simulink model "rigidBody2d03v"  (Simulink 7.5)
settings: Solver=ode45  StartTime=0.0  StopTime=2  RelTol=1e-4
values from neighbouring files (symbols this model uses):
  c = 1000    [runModel03v.m]    (also in runModel04v.m = 5000)
  dy = 0    [runModel03v.m]    (also in runModel04v.m)
  dyt1 = .2    (= 0.2)    [runModel03v.m]    (also in runModel04v.m = 1000)
  dyt2 = .2 + L/v0    (= 0.231666666667)    [runModel03v.m]    (also in runModel04v.m = 1000)
  FB1t = .2    (= 0.2)    [runModel03v.m]
  FB1x = -1600    [runModel03v.m]
  FB2 = [-1600 0]    [runModel03v.m]
  FD = [-645 0]    [runModel03v.m]    (also in runModel04v.m)
  FE1 = [120 0]    [runModel03v.m]    (also in runModel04v.m)
  FE2t = 1000    [runModel03v.m]    (also in runModel04v.m = 10000)
  FE2x = 120    [runModel03v.m]    (also in runModel04v.m)
  I = 1/4*m*R^2 + 1/12*m*L^2    (= 405.066666667)    [runModel03v.m]    (also in runModel04v.m)
  k = 111000*2    (= 222000)    [runModel03v.m]    (also in runModel04v.m)
  L = 3.8    [runModel03v.m]    (also in runModel04v.m)
  m = 320    [runModel03v.m]    (also in runModel04v.m)
  rB1 = [0 0.5]    [runModel03v.m]    (also in runModel04v.m)
  rB2 = [0 -0.5]    [runModel03v.m]    (also in runModel04v.m)
  rDx = 0    [runModel03v.m]    (also in runModel04v.m)
  rE1 = [0 0.5]    [runModel03v.m]    (also in runModel04v.m)
  rE2 = [0 -0.5]    [runModel03v.m]    (also in runModel04v.m)
  rS1 = [-1.9 0]    [runModel03v.m]    (also in runModel04v.m)
  rS2 = [1.9 0]    [runModel03v.m]    (also in runModel04v.m)
  v0 = 120    [runModel03v.m]    (also in runModel04v.m)
settings Model: Creator=aaron  LastModifiedBy=aaron
settings DebuggingCC: SolverPrmCheckMsg=none

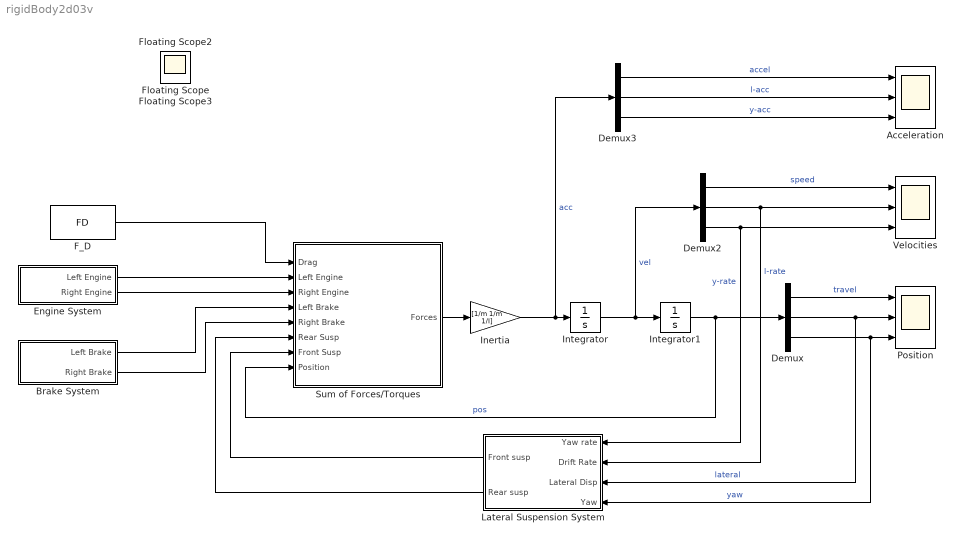
== system rigidBody2d03v ==
  Acceleration : Scope  NumInputPorts=3
      settings: TimeRange=2  YMin=1~-1~-1  YMax=3.5~1~1  SaveName=position3
  Brake System : Subsystem
  Demux : Demux  Outputs=3
  Demux2 : Demux  Outputs=3
  Demux3 : Demux  Outputs=3
  Engine System : Subsystem
  F_D : Constant  Value=FD  OutDataType=fixdt(1, 16)  OutScaling=2^0
  Inertia : Gain  Gain=[1/m 1/m 1/I]  ParameterDataType=fixdt(1, 16)  ParameterScaling=2^0  OutDataType=fixdt(1, 16)  OutScaling=2^0
  Integrator : Integrator  InitialCondition=[v0 0 0]
  Integrator1 : Integrator  InitialCondition=[0 0 0]
  Lateral Suspension System : Subsystem
  Position : Scope  NumInputPorts=3
      settings: YMin=-1.5e+007~-52.5~-0.7  YMax=0~2.5~0.05  SaveName=position
  Sum of Forces/Torques : Subsystem
  Velocities : Scope  NumInputPorts=3
      settings: YMin=-5~-5~-5  YMax=5~5~5  SaveName=position2
  Floating Scope : Scope
      settings: Floating=on
  Floating Scope2 : Scope
      settings: Floating=on  SaveName=ScopeData2
  Floating Scope3 : Scope
      settings: Floating=on  SaveName=ScopeData3
  wires:
  Integrator/1 -> Integrator1/1, Demux2/1  "vel"
  Inertia/1 -> Demux3/1, Integrator/1  "acc"
  Sum of Forces/Torques/1(Forces) -> Inertia/1
  Integrator1/1 -> Demux/1, Sum of Forces/Torques/8(Position)  "pos"
  Demux/1 -> Position/1  "travel"
  Demux/2 -> Position/2, Lateral Suspension System/3(Lateral Disp)  "lateral"
  Demux/3 -> Position/3, Lateral Suspension System/4(Yaw)  "yaw"
  Demux2/1 -> Velocities/1  "speed"
  Demux2/2 -> Velocities/2, Lateral Suspension System/2(Drift Rate)  "l-rate"
  Demux2/3 -> Velocities/3, Lateral Suspension System/1(Yaw rate)  "y-rate"
  Demux3/1 -> Acceleration/1  "accel"
  Demux3/2 -> Acceleration/2  "l-acc"
  Demux3/3 -> Acceleration/3  "y-acc"
  Engine System/1(Left Engine) -> Sum of Forces/Torques/2(Left Engine)
  Lateral Suspension System/1(Front susp) -> Sum of Forces/Torques/7(Front Susp)
  Lateral Suspension System/2(Rear susp) -> Sum of Forces/Torques/6(Rear Susp)
  F_D/1 -> Sum of Forces/Torques/1(Drag)
  Engine System/2(Right Engine) -> Sum of Forces/Torques/3(Right Engine)
  Brake System/1(Left Brake) -> Sum of Forces/Torques/4(Left Brake)
  Brake System/2(Right Brake) -> Sum of Forces/Torques/5(Right Brake)

== system rigidBody2d03v/Brake System ==
  F_B1y : Constant  Value=0  OutDataType=fixdt(1, 16)  OutScaling=2^0
  F_B2 : Constant  Value=FB2  OutDataType=fixdt(1, 16)  OutScaling=2^0
  Mux : Mux  Inputs=2
  Step : Step  Time=FB1t  Before=FB1x  After=0  SampleTime=0
  Left Brake : Outport
  Right Brake : Outport  Port=2
  wires:
  Step/1 -> Mux/1  "forceX"
  F_B1y/1 -> Mux/2  "forceY"
  F_B2/1 -> Right Brake/1
  Mux/1 -> Left Brake/1

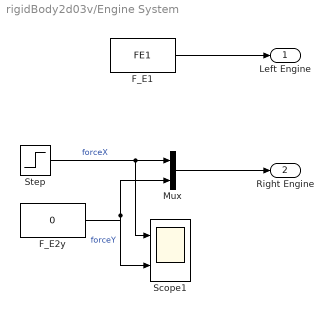
== system rigidBody2d03v/Engine System ==
  F_E1 : Constant  Value=FE1  OutDataType=fixdt(1, 16)  OutScaling=2^0
  F_E2y : Constant  Value=0  OutDataType=fixdt(1, 16)  OutScaling=2^0
  Mux : Mux  Inputs=2
  Scope1 : Scope  NumInputPorts=2
      settings: YMin=-5~-5  YMax=5~5  SaveName=engineErr
  Step : Step  Time=FE2t  Before=FE2x  After=0  SampleTime=0
  Left Engine : Outport
  Right Engine : Outport  Port=2
  wires:
  Step/1 -> Mux/1, Scope1/1  "forceX"
  F_E2y/1 -> Mux/2, Scope1/2  "forceY"
  F_E1/1 -> Left Engine/1
  Mux/1 -> Right Engine/1

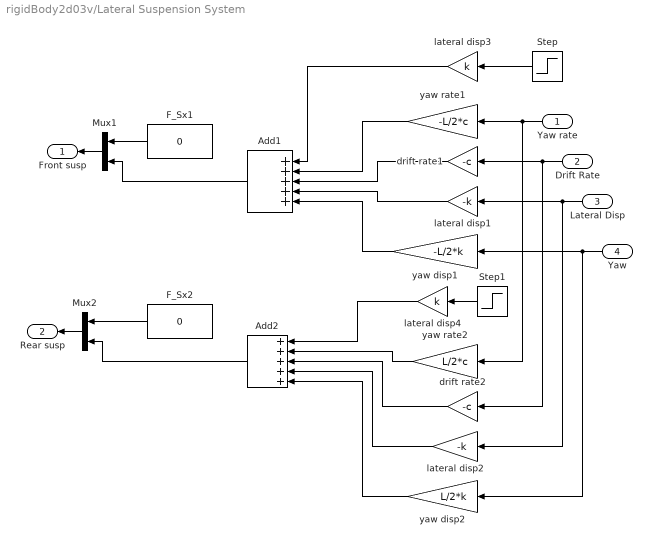
== system rigidBody2d03v/Lateral Suspension System ==
  Yaw rate : Inport
  Drift Rate : Inport  Port=2
  Lateral Disp : Inport  Port=3
  Yaw : Inport  Port=4
  Add1 : Sum  Inputs=+++++  OutDataType=fixdt(1, 16)  OutScaling=2^-10
  Add2 : Sum  Inputs=+++++  OutDataType=fixdt(1, 16)  OutScaling=2^-10
  F_Sx1 : Constant  Value=0  OutDataType=fixdt(1, 16)  OutScaling=2^0
  F_Sx2 : Constant  Value=0  OutDataType=fixdt(1, 16)  OutScaling=2^0
  Mux1 : Mux  Inputs=2
  Mux2 : Mux  Inputs=2
  Step : Step  Time=dyt1  After=dy  SampleTime=0
  Step1 : Step  Time=dyt2  After=dy  SampleTime=0
  drift rate1 : Gain  Gain=-c  ParameterDataType=fixdt(1, 16)  ParameterScaling=2^0  OutDataType=fixdt(1, 16)  OutScaling=2^0
  drift rate2 : Gain  Gain=-c  ParameterDataType=fixdt(1, 16)  ParameterScaling=2^0  OutDataType=fixdt(1, 16)  OutScaling=2^0
  lateral disp1 : Gain  Gain=-k  ParameterDataType=fixdt(1, 16)  ParameterScaling=2^0  OutDataType=fixdt(1, 16)  OutScaling=2^0
  lateral disp2 : Gain  Gain=-k  ParameterDataType=fixdt(1, 16)  ParameterScaling=2^0  OutDataType=fixdt(1, 16)  OutScaling=2^0
  lateral disp3 : Gain  Gain=k  ParameterDataType=fixdt(1, 16)  ParameterScaling=2^0  OutDataType=fixdt(1, 16)  OutScaling=2^0
  lateral disp4 : Gain  Gain=k  ParameterDataType=fixdt(1, 16)  ParameterScaling=2^0  OutDataType=fixdt(1, 16)  OutScaling=2^0
  yaw disp1 : Gain  Gain=-L/2*k  ParameterDataType=fixdt(1, 16)  ParameterScaling=2^0  OutDataType=fixdt(1, 16)  OutScaling=2^0
  yaw disp2 : Gain  Gain=L/2*k  ParameterDataType=fixdt(1, 16)  ParameterScaling=2^0  OutDataType=fixdt(1, 16)  OutScaling=2^0
  yaw rate1 : Gain  Gain=-L/2*c  ParameterDataType=fixdt(1, 16)  ParameterScaling=2^0  OutDataType=fixdt(1, 16)  OutScaling=2^0
  yaw rate2 : Gain  Gain=L/2*c  ParameterDataType=fixdt(1, 16)  ParameterScaling=2^0  OutDataType=fixdt(1, 16)  OutScaling=2^0
  Front susp : Outport
  Rear susp : Outport  Port=2
  wires:
  F_Sx1/1 -> Mux1/1
  Add1/1 -> Mux1/2
  F_Sx2/1 -> Mux2/1
  Add2/1 -> Mux2/2
  lateral disp1/1 -> Add1/4
  lateral disp2/1 -> Add2/4
  drift rate2/1 -> Add2/3
  drift rate1/1 -> Add1/3
  yaw disp2/1 -> Add2/5
  yaw disp1/1 -> Add1/5
  yaw rate2/1 -> Add2/2
  yaw rate1/1 -> Add1/2
  Yaw rate/1 -> yaw rate1/1, yaw rate2/1
  Drift Rate/1 -> drift rate1/1, drift rate2/1
  Lateral Disp/1 -> lateral disp1/1, lateral disp2/1
  Yaw/1 -> yaw disp1/1, yaw disp2/1
  Mux1/1 -> Front susp/1
  Mux2/1 -> Rear susp/1
  Step/1 -> lateral disp3/1
  lateral disp3/1 -> Add1/1
  Step1/1 -> lateral disp4/1
  lateral disp4/1 -> Add2/1

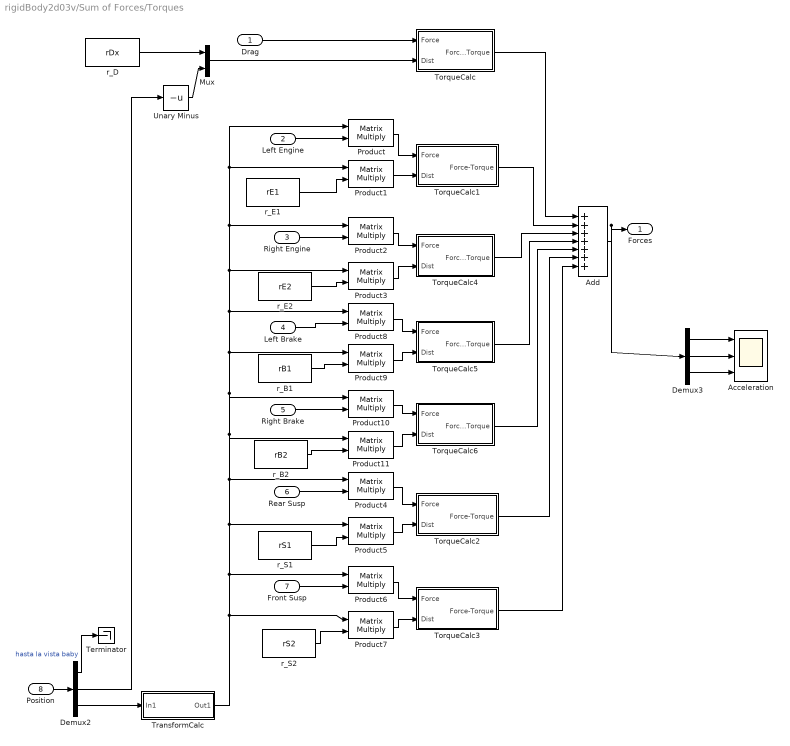
== system rigidBody2d03v/Sum of Forces/Torques ==
  Drag : Inport
  Left Engine : Inport  Port=2
  Right Engine : Inport  Port=3
  Left Brake : Inport  Port=4
  Right Brake : Inport  Port=5
  Rear Susp : Inport  Port=6
  Front Susp : Inport  Port=7
  Position : Inport  Port=8
  Acceleration : Scope  NumInputPorts=3
      settings: YMin=-5~-5~-5  YMax=5~5~5  SaveName=position1
  Add : Sum  Inputs=+++++++  OutDataType=fixdt(1, 16)  OutScaling=2^-10
  Demux2 : Demux  Outputs=3
  Demux3 : Demux  Outputs=3
  Mux : Mux  Inputs=2
  Product{,1..11} (12 alike) : Product  Multiplication=Matrix(*)  OutDataType=fixdt(1, 16)  OutScaling=2^0  RndMeth=Zero
  Terminator : Terminator
  TorqueCalc : Subsystem
  TorqueCalc1 : Subsystem
  TorqueCalc2 : Subsystem
  TorqueCalc3 : Subsystem
  TorqueCalc4 : Subsystem
  TorqueCalc5 : Subsystem
  TorqueCalc6 : Subsystem
  TransformCalc : Subsystem
  Unary Minus : UnaryMinus
  r_B1 : Constant  Value=rB1  OutDataType=fixdt(1, 16)  OutScaling=2^0
  r_B2 : Constant  Value=rB2  OutDataType=fixdt(1, 16)  OutScaling=2^0
  r_D : Constant  Value=rDx  OutDataType=fixdt(1, 16)  OutScaling=2^0
  r_E1 : Constant  Value=rE1  OutDataType=fixdt(1, 16)  OutScaling=2^0
  r_E2 : Constant  Value=rE2  OutDataType=fixdt(1, 16)  OutScaling=2^0
  r_S1 : Constant  Value=rS1  OutDataType=fixdt(1, 16)  OutScaling=2^0
  r_S2 : Constant  Value=rS2  OutDataType=fixdt(1, 16)  OutScaling=2^0
  Forces : Outport
  wires:
  Drag/1 -> TorqueCalc/1(Force)
  Add/1 -> Forces/1, Demux3/1
  TorqueCalc1/1(Force-Torque) -> Add/2
  TorqueCalc/1(Force-Torque) -> Add/1
  TorqueCalc4/1(Force-Torque) -> Add/3
  Position/1 -> Demux2/1
  Demux2/3 -> TransformCalc/1(In1)
  Left Engine/1 -> Product/2
  TransformCalc/1(Out1) -> Product4/1, Product/1, Product1/1, Product2/1, Product3/1, Product8/1, Product9/1, Product10/1, Product11/1, Product5/1, Product6/1, Product7/1
  Right Engine/1 -> Product2/2
  r_E1/1 -> Product1/2
  r_E2/1 -> Product3/2
  Product/1 -> TorqueCalc1/1(Force)
  Product1/1 -> TorqueCalc1/2(Dist)
  Product2/1 -> TorqueCalc4/1(Force)
  Product3/1 -> TorqueCalc4/2(Dist)
  Product4/1 -> TorqueCalc2/1(Force)
  Product5/1 -> TorqueCalc2/2(Dist)
  Product6/1 -> TorqueCalc3/1(Force)
  Product7/1 -> TorqueCalc3/2(Dist)
  Rear Susp/1 -> Product4/2
  r_S1/1 -> Product5/2
  Front Susp/1 -> Product6/2
  r_S2/1 -> Product7/2
  Demux3/1 -> Acceleration/1
  Demux3/2 -> Acceleration/2
  Demux3/3 -> Acceleration/3
  r_D/1 -> Mux/1
  Unary Minus/1 -> Mux/2
  Mux/1 -> TorqueCalc/2(Dist)
  Left Brake/1 -> Product8/2
  Product8/1 -> TorqueCalc5/1(Force)
  r_B1/1 -> Product9/2
  Right Brake/1 -> Product10/2
  r_B2/1 -> Product11/2
  Product11/1 -> TorqueCalc6/2(Dist)
  Product10/1 -> TorqueCalc6/1(Force)
  Product9/1 -> TorqueCalc5/2(Dist)
  TorqueCalc3/1(Force-Torque) -> Add/7
  TorqueCalc2/1(Force-Torque) -> Add/6
  TorqueCalc6/1(Force-Torque) -> Add/5
  TorqueCalc5/1(Force-Torque) -> Add/4
  Demux2/1 -> Terminator/1  "hasta la vista baby"
  Demux2/2 -> Unary Minus/1

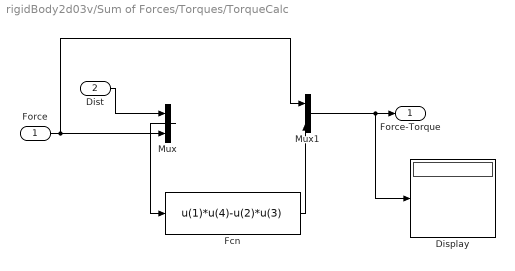
== system rigidBody2d03v/Sum of Forces/Torques/TorqueCalc ==
  Force : Inport
  Dist : Inport  Port=2
  Display : Display
  Fcn : Fcn  Expr=u(1)*u(4)-u(2)*u(3)
  Mux : Mux  Inputs=2
  Mux1 : Mux  Inputs=2
  Force-Torque : Outport
  wires:
  Force/1 -> Mux1/1, Mux/2
  Mux/1 -> Fcn/1
  Fcn/1 -> Mux1/2
  Mux1/1 -> Display/1, Force-Torque/1
  Dist/1 -> Mux/1

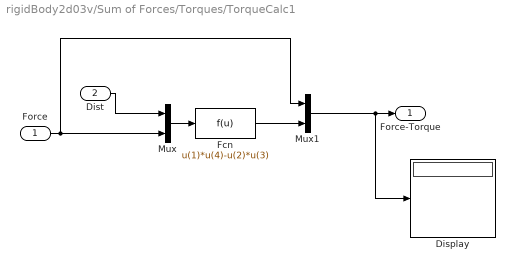
== system rigidBody2d03v/Sum of Forces/Torques/TorqueCalc1 ==
  Force : Inport
  Dist : Inport  Port=2
  Display : Display
  Fcn : Fcn  Expr=u(1)*u(4)-u(2)*u(3)
  Mux : Mux  Inputs=2
  Mux1 : Mux  Inputs=2
  Force-Torque : Outport
  wires:
  Force/1 -> Mux1/1, Mux/2
  Mux/1 -> Fcn/1
  Fcn/1 -> Mux1/2
  Mux1/1 -> Display/1, Force-Torque/1
  Dist/1 -> Mux/1

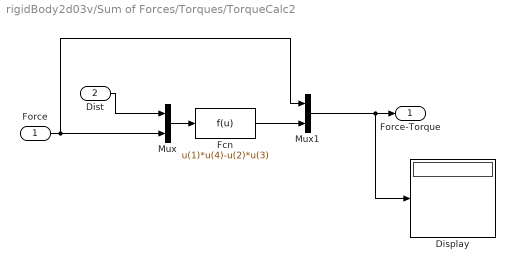
== system rigidBody2d03v/Sum of Forces/Torques/TorqueCalc2 ==
  Force : Inport
  Dist : Inport  Port=2
  Display : Display
  Fcn : Fcn  Expr=u(1)*u(4)-u(2)*u(3)
  Mux : Mux  Inputs=2
  Mux1 : Mux  Inputs=2
  Force-Torque : Outport
  wires:
  Force/1 -> Mux1/1, Mux/2
  Mux/1 -> Fcn/1
  Fcn/1 -> Mux1/2
  Mux1/1 -> Display/1, Force-Torque/1
  Dist/1 -> Mux/1

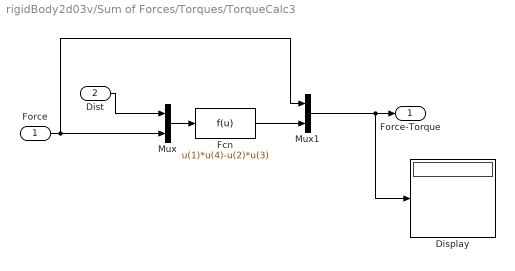
== system rigidBody2d03v/Sum of Forces/Torques/TorqueCalc3 ==
  Force : Inport
  Dist : Inport  Port=2
  Display : Display
  Fcn : Fcn  Expr=u(1)*u(4)-u(2)*u(3)
  Mux : Mux  Inputs=2
  Mux1 : Mux  Inputs=2
  Force-Torque : Outport
  wires:
  Force/1 -> Mux1/1, Mux/2
  Mux/1 -> Fcn/1
  Fcn/1 -> Mux1/2
  Mux1/1 -> Display/1, Force-Torque/1
  Dist/1 -> Mux/1

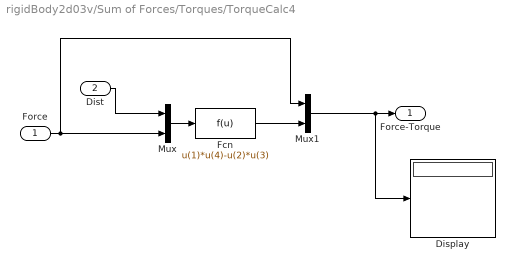
== system rigidBody2d03v/Sum of Forces/Torques/TorqueCalc4 ==
  Force : Inport
  Dist : Inport  Port=2
  Display : Display
  Fcn : Fcn  Expr=u(1)*u(4)-u(2)*u(3)
  Mux : Mux  Inputs=2
  Mux1 : Mux  Inputs=2
  Force-Torque : Outport
  wires:
  Force/1 -> Mux1/1, Mux/2
  Mux/1 -> Fcn/1
  Fcn/1 -> Mux1/2
  Mux1/1 -> Display/1, Force-Torque/1
  Dist/1 -> Mux/1

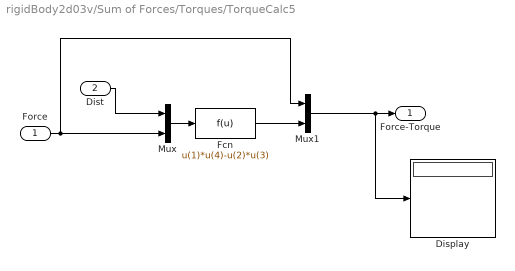
== system rigidBody2d03v/Sum of Forces/Torques/TorqueCalc5 ==
  Force : Inport
  Dist : Inport  Port=2
  Display : Display
  Fcn : Fcn  Expr=u(1)*u(4)-u(2)*u(3)
  Mux : Mux  Inputs=2
  Mux1 : Mux  Inputs=2
  Force-Torque : Outport
  wires:
  Force/1 -> Mux1/1, Mux/2
  Mux/1 -> Fcn/1
  Fcn/1 -> Mux1/2
  Mux1/1 -> Display/1, Force-Torque/1
  Dist/1 -> Mux/1

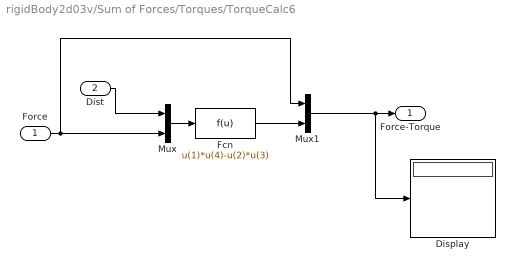
== system rigidBody2d03v/Sum of Forces/Torques/TorqueCalc6 ==
  Force : Inport
  Dist : Inport  Port=2
  Display : Display
  Fcn : Fcn  Expr=u(1)*u(4)-u(2)*u(3)
  Mux : Mux  Inputs=2
  Mux1 : Mux  Inputs=2
  Force-Torque : Outport
  wires:
  Force/1 -> Mux1/1, Mux/2
  Mux/1 -> Fcn/1
  Fcn/1 -> Mux1/2
  Mux1/1 -> Display/1, Force-Torque/1
  Dist/1 -> Mux/1

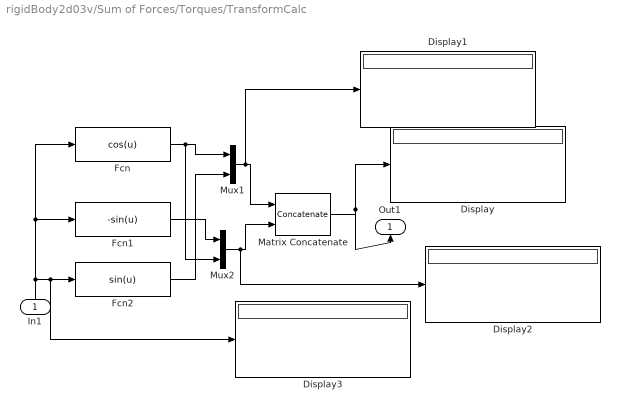
== system rigidBody2d03v/Sum of Forces/Torques/TransformCalc ==
  In1 : Inport
  Display{,1..3} (4 alike) : Display
  Fcn : Fcn  Expr=cos(u)
  Fcn1 : Fcn  Expr=-sin(u)
  Fcn2 : Fcn  Expr=sin(u)
  Matrix Concatenate : Concatenate  Mode=Multidimensional array  ConcatenateDimension=2
  Mux1 : Mux  Inputs=2
  Mux2 : Mux  Inputs=2
  Out1 : Outport
  wires:
  In1/1 -> Fcn/1, Fcn1/1, Fcn2/1, Display3/1
  Fcn/1 -> Mux1/1, Mux2/2
  Mux2/1 -> Matrix Concatenate/2, Display2/1
  Mux1/1 -> Matrix Concatenate/1, Display1/1
  Fcn2/1 -> Mux1/2
  Fcn1/1 -> Mux2/1
  Matrix Concatenate/1 -> Display/1, Out1/1
